simulink model "Laboratory_1_Simulink_1"  (R2023b)
settings: Solver=FixedStepDiscrete  StartTime=0.0  StopTime=10.0  FixedStep=0.5  RelTol=1e-3
settings Model: Creator=cosmi  LastModifiedBy=cosmi

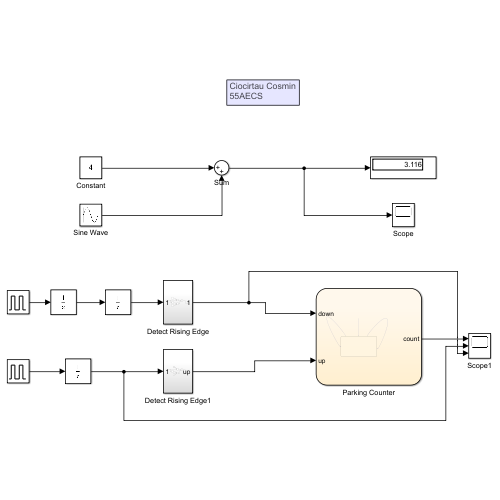
[thumbnail: Simulink's stored preview of the top-level diagram]
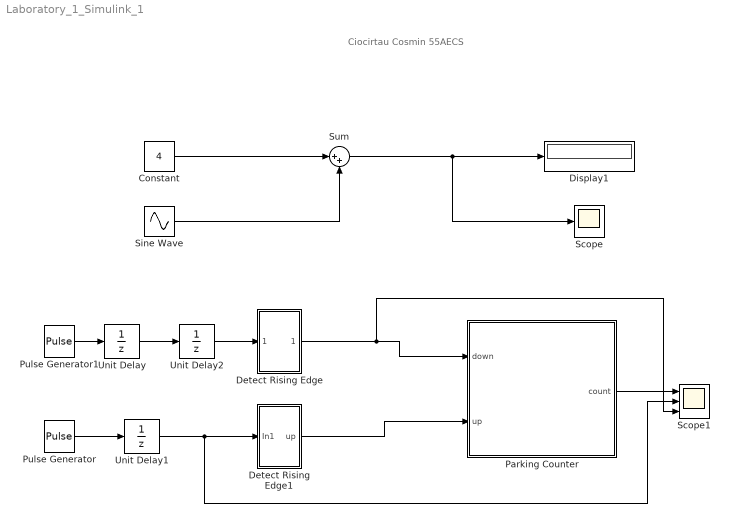
== system Laboratory_1_Simulink_1 ==
  note: Ciocirtau Cosmin
      | 55AECS
  Constant : Constant  Value=4
  Detect Rising Edge : Subsystem
  Detect Rising Edge1 : Subsystem
  Display1 : Display
  Parking Counter : Stateflow chart  TreatAsAtomicUnit=on
  Pulse Generator : DiscretePulseGenerator  PulseType=Time based  Period=4  PulseWidth=50
  Pulse Generator1 : DiscretePulseGenerator  PulseType=Time based  Period=4  PulseWidth=50
  Scope : Scope
  Scope1 : Scope  NumInputPorts=3
  Sine Wave : Sin  Amplitude=1.5  Frequency=3  Phase=pi/4  SampleTime=0
  Sum : Sum  Inputs=|++
  Unit Delay : UnitDelay  SampleTime=-1  HasFrameUpgradeWarning=on
  Unit Delay1 : UnitDelay  SampleTime=-1  HasFrameUpgradeWarning=on
  Unit Delay2 : UnitDelay  SampleTime=-1  HasFrameUpgradeWarning=on
  wires:
  Constant/1 -> Sum/1
  Sine Wave/1 -> Sum/2
  Sum/1 -> Scope/1, Display1/1
  Parking Counter/1(count) -> Scope1/1
  Detect Rising Edge/1(Out1) -> Scope1/3, Parking Counter/1(down)
  Detect Rising Edge1/1(up) -> Parking Counter/2(up)
  Unit Delay1/1 -> Detect Rising Edge1/1(In1), Scope1/2
  Pulse Generator/1 -> Unit Delay1/1
  Pulse Generator1/1 -> Unit Delay/1
  Unit Delay/1 -> Unit Delay2/1
  Unit Delay2/1 -> Detect Rising Edge/1(In1)

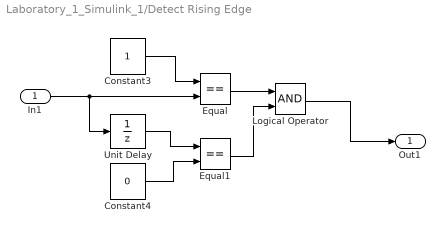
== system Laboratory_1_Simulink_1/Detect Rising Edge ==
  In1 : Inport
  Constant3 : Constant  OutDataTypeStr=boolean
  Constant4 : Constant  Value=0  OutDataTypeStr=boolean
  Equal : RelationalOperator  Operator===  OutDataTypeStr=boolean  RndMeth=Simplest  InputSameDT=off
  Equal1 : RelationalOperator  Operator===  OutDataTypeStr=boolean  RndMeth=Simplest  InputSameDT=off
  Logical Operator : Logic  AllPortsSameDT=off  OutDataTypeStr=boolean
  Unit Delay : UnitDelay  SampleTime=-1  HasFrameUpgradeWarning=on
  Out1 : Outport
  wires:
  Constant4/1 -> Equal1/2
  In1/1 -> Equal/2, Unit Delay/1
  Constant3/1 -> Equal/1
  Equal/1 -> Logical Operator/1
  Equal1/1 -> Logical Operator/2
  Unit Delay/1 -> Equal1/1
  Logical Operator/1 -> Out1/1

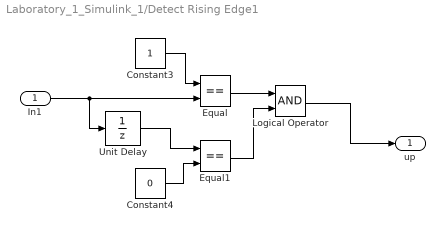
== system Laboratory_1_Simulink_1/Detect Rising Edge1 ==
  In1 : Inport
  Constant3 : Constant  OutDataTypeStr=boolean
  Constant4 : Constant  Value=0  OutDataTypeStr=boolean
  Equal : RelationalOperator  Operator===  OutDataTypeStr=boolean  RndMeth=Simplest  InputSameDT=off
  Equal1 : RelationalOperator  Operator===  OutDataTypeStr=boolean  RndMeth=Simplest  InputSameDT=off
  Logical Operator : Logic  AllPortsSameDT=off  OutDataTypeStr=boolean
  Unit Delay : UnitDelay  SampleTime=-1  HasFrameUpgradeWarning=on
  up : Outport
  wires:
  Constant4/1 -> Equal1/2
  In1/1 -> Equal/2, Unit Delay/1
  Constant3/1 -> Equal/1
  Equal/1 -> Logical Operator/1
  Equal1/1 -> Logical Operator/2
  Unit Delay/1 -> Equal1/1
  Logical Operator/1 -> up/1

== stateflow chart Laboratory_1_Simulink_1/Parking Counter ==
  state ParkingState
  ParkingState -> ParkingState [order 2] : [up==false && down==true && count>0]/
      | {count=count-1;}
  ParkingState -> ParkingState [order 1] : [(up==true) && (down==false) && (count<10)]/
      | {count=count+1;}
  (default) -> ParkingState : {count=0;}
  data: down input; up input boolean; count output =0
